simulink model "VCMGCM1962020b_v2"  (R2020b)
settings: Solver=FixedStepDiscrete  StartTime=0.0  StopTime=10.0  FixedStep=0.005  RelTol=1e-3  EnableMultiTasking=on
PreLoadFcn:
  | try, model_open; catch, disp('Error occurred while executing model pre-load callback: model_open.m'); disp('Please assure that the MATLAB working directory is set to the model directory before opening.'); end
InitFcn:
  | try, model_open; catch, end
undefined symbols (not defined in the file): Bridge, GCM, H, raptor_get_param_eval, raptor_get_safe_string, raptor_xcp_function
libraries: Blocks_lib x1165, Raptor_lib x665, simulink x62, VCM_lib x5
(part 21 of 23)

== system VCMGCM1962020b_v2/Fgnd/Control/Drive Inverter/Motor Torque Request/Driver Torque Request/Cruise Control/Setpoint ==
  Data : Inport
  Bus Creator : BusCreator  Inputs=3
  Bus Selector5 : BusSelector  OutputSignals=VirtualSensors.Spd.VehSpd [kph],VirtualSensors.Driver.CCOn [Bool],VirtualSensors.Driver.CCSetCst [Bool],VirtualSensors.Driver.CCRsmAcc [Bool]
  Enable : Subsystem
  Header : Blocks_lib/Header  width=Portrait  addtext=''
  Meas&Ovrd : Blocks_lib/Meas&Ovrd  nam='CCActv'  name_source=Parameter  view_as=Number  enum_struct={}  gain=1  min=-inf  max=inf  precision=''  units='Bool'  help='Cruise control active'  group=group
  Meas&Ovrd1 : Blocks_lib/Meas&Ovrd  nam='CCSetpt'  name_source=Parameter  view_as=Number  enum_struct={}  gain=1  min=-inf  max=inf  precision=''  units='kph'  help='Cruise control setpoint'  group=group
  Setpoint : Stateflow chart  TreatAsAtomicUnit=on
  SetptMnMx : Subsystem
  Standby : Subsystem
  raptor_adjustment : Raptor_lib/Data Storage/raptor_adjustment  paramName='CCTapTimeThr'  nameSource=Parameter  initValue=0 / samptime  dataType=uint16  storage=Calibration  calDispType=Number  calEnum={'Disabled', 'Enabled'}  calGain=samptime  calOffset=0  calMax=inf  calMin=-inf  calFormat=''  calUnit='sec'  calHelp='Cruise control tap time threshold'  calAccess=1  calFunction=group  calDispHeaders=off  calColHeaders={'Col1' 'Col2' 'Col3'}  calRowHeaders={'Row1' 'Row2' 'Row3'}
      settings: SourceProductName=Raptor
  raptor_adjustment1 : Raptor_lib/Data Storage/raptor_adjustment  paramName='CCDecDeltaMx'  nameSource=Parameter  initValue=0  dataType=double  storage=Calibration  calDispType=Number  calEnum={'Disabled', 'Enabled'}  calGain=1  calOffset=0  calMax=inf  calMin=-inf  calFormat=''  calUnit='kph'  calHelp='Cruise control decrement delta (between vehicle speed and setpoint) maximum'  calAccess=1  calFunction=group  calDispHeaders=off  calColHeaders={'Col1' 'Col2' 'Col3'}  calRowHeaders={'Row1' 'Row2' 'Row3'}
      settings: SourceProductName=Raptor
  raptor_adjustment2 : Raptor_lib/Data Storage/raptor_adjustment  paramName='CCTapInc'  nameSource=Parameter  initValue=0  dataType=double  storage=Calibration  calDispType=Number  calEnum={'Disabled', 'Enabled'}  calGain=1  calOffset=0  calMax=inf  calMin=-inf  calFormat=''  calUnit='kph'  calHelp='Cruise control tap increment'  calAccess=1  calFunction=group  calDispHeaders=off  calColHeaders={'Col1' 'Col2' 'Col3'}  calRowHeaders={'Row1' 'Row2' 'Row3'}
      settings: SourceProductName=Raptor
  raptor_adjustment3 : Raptor_lib/Data Storage/raptor_adjustment  paramName='CCAccRate'  nameSource=Parameter  initValue=0 * samptime  dataType=double  storage=Calibration  calDispType=Number  calEnum={'Disabled', 'Enabled'}  calGain=1/samptime  calOffset=0  calMax=inf  calMin=-inf  calFormat=''  calUnit='kph/s'  calHelp='Cruise control accelerate rate'  calAccess=1  calFunction=group  calDispHeaders=off  calColHeaders={'Col1' 'Col2' 'Col3'}  calRowHeaders={'Row1' 'Row2' 'Row3'}
      settings: SourceProductName=Raptor
  raptor_measurement : Raptor_lib/Data Storage/raptor_measurement  paramName='CCState'  nameSource=Parameter  calDispType=Number  calEnum={}  calGain=1  calOffset=0  calMax=inf  calMin=-inf  calFormat=''  calUnit='enum'  calHelp='Cruise control state'  calAccess=1  calFunction=group  calVisible=on
      settings: SourceProductName=Raptor
  Setpt : Outport  VectorParamsAs1DForOutWhenUnconnected=off
  wires:
  SetptMnMx/2(Mn) -> Setpoint/12(SetptMn)
  SetptMnMx/1(Mx) -> Setpoint/11(SetptMx)
  Setpoint/1(State) -> Bus Creator/1, raptor_measurement/1  "CCState [enum]"
  Meas&Ovrd1/1 -> Bus Creator/3
  Meas&Ovrd/1 -> Bus Creator/2
  raptor_adjustment1/1 -> Setpoint/8(DecDeltaMx)
  raptor_adjustment2/1 -> Setpoint/9(TapInc)
  Bus Creator/1 -> Setpt/1  "CCSetpt"
  Setpoint/2(Actv) -> Meas&Ovrd/1
  Setpoint/3(Setpt) -> Meas&Ovrd1/1
  raptor_adjustment/1 -> Setpoint/7(TapThr)
  Enable/1(Enbl) -> Setpoint/1(Enbl)
  raptor_adjustment3/1 -> Setpoint/10(AccInc)
  Standby/1(Stndby) -> Setpoint/2(Standby)
  Bus Selector5/2 -> Setpoint/4(On)  "<CCOn [Bool]>"
  Bus Selector5/3 -> Setpoint/5(SetCst)  "<CCSetCst [Bool]>"
  Bus Selector5/4 -> Setpoint/6(RsmAcc)  "<CCRsmAcc [Bool]>"
  Data/1 -> Enable/1(Data), Standby/1(Data), Bus Selector5/1, SetptMnMx/1(Data)
  Bus Selector5/1 -> Setpoint/3(Spd)  "<VehSpd [kph]>"

== system VCMGCM1962020b_v2/Fgnd/Control/Drive Inverter/Motor Torque Request/Driver Torque Request/Driveability/Rate Limit ==
  Data : Inport
  TrqReq : Inport  Port=2
  Bus Selector : BusSelector  OutputSignals=VirtualSensors.Spd.VehSpd [kph]
  Compare To Zero : simulink/Logic and Bit Operations/Compare To Zero  relop=<  OutDataTypeStr=boolean
  Gain : Gain  Gain=-1
  Header : Blocks_lib/Header  width=Portrait  addtext=''
  Multiport Switch : MultiPortSwitch  DataPortOrder=Zero-based contiguous  Inputs=2  zeroidx=on  InputSameDT=on
  Mux : Mux  Inputs=2
  Selector : Selector  InputPortWidth=2  IndexOptions=Index vector (dialog)  Indices=[2 1]  OutputSizes=1
  raptor_table_axis : Raptor_lib/Table Lookup/raptor_table_axis  dataName='VehSpd05IdxArr'  initValue=[1:05]  dataType=double  storage=Calibration  calVisible=on  calGain=1.0  calOffset=0  calMax=Inf  calMin=-Inf  calFormat='-1'  calUnit='kph'  calHelp='Index array'  calAccess=1  calFunction=group
      settings: SourceProductName=Raptor
  raptor_table_interpolate_1d : Raptor_lib/Table Lookup/raptor_table_interpolate_1d  dataName='DrvTrqReqRateLimIncTbl'  initValue=zeros(1,5)  dataType=double  storage=Calibration  adapt=off  adaptMode=Adapt between points  adaptOut=off  calVisible=on  calGain=1.0  calOffset=0.0  calMax=Inf  calMin=-Inf  calFormat='-1'  calUnit='Nm/s'  calHelp='Driver torque request rate limit (in increasing direction away from zero)'  calAccess=1  calFunction=group  measureEnable=on  mName='DrvTrqReqRateLimInc'
      settings: SourceProductName=Raptor
  raptor_table_interpolate_1d1 : Raptor_lib/Table Lookup/raptor_table_interpolate_1d  dataName='DrvTrqReqRateLimDecTbl'  initValue=zeros(1,5)  dataType=double  storage=Calibration  adapt=off  adaptMode=Adapt between points  adaptOut=off  calVisible=on  calGain=1.0  calOffset=0.0  calMax=Inf  calMin=-Inf  calFormat='-1'  calUnit='Nm/s'  calHelp='Driver torque request rate limit (in decreasing direction towards zero)'  calAccess=1  calFunction=group  measureEnable=on  mName='DrvTrqReqRateLimDec'
      settings: SourceProductName=Raptor
  Nm/s : Outport  VectorParamsAs1DForOutWhenUnconnected=off
  wires:
  Multiport Switch/1 -> Nm/s/1
  raptor_table_interpolate_1d1/1 -> Mux/2
  raptor_table_interpolate_1d/1 -> Mux/1
  Gain/1 -> Multiport Switch/3
  Selector/1 -> Gain/1
  Compare To Zero/1 -> Multiport Switch/1
  Data/1 -> Bus Selector/1
  Bus Selector/1 -> raptor_table_axis/1  "<VehSpd [kph]>"
  TrqReq/1 -> Compare To Zero/1
  raptor_table_axis/1 -> raptor_table_interpolate_1d/1, raptor_table_interpolate_1d1/1
  Mux/1 -> Selector/1, Multiport Switch/2

== system VCMGCM1962020b_v2/Fgnd/Control/Drive Inverter/Motor Torque Request/Driver Torque Request/Pedal Torque Request/APP When Two Pedal Driving ==
  Data : Inport
  Bus Selector : BusSelector  OutputSignals=VirtualSensors.Driver.BrkSw [Bool],VirtualSensors.Driver.APP [%]
  Header : Blocks_lib/Header  width=Portrait  addtext=''
  MinMax : MinMax  Inputs=2
  Multiport Switch : MultiPortSwitch  DataPortOrder=Zero-based contiguous  Inputs=2  zeroidx=on
  raptor_adjustment : Raptor_lib/Data Storage/raptor_adjustment  paramName='APPMxTwoPedalDrv'  nameSource=Parameter  initValue=0  dataType=double  storage=Calibration  calDispType=Number  calEnum={'False', 'True'}  calGain=1.0  calOffset=0.0  calMax=inf  calMin=-inf  calFormat='-1'  calUnit='%'  calHelp='APP maximum (when two pedal driving)'  calAccess=1  calFunction=group  calDispHeaders=off  calColHeaders={'Col1' 'Col2' 'Col3'}  calRowHeaders={'Row1' 'Row2' 'Row3'}
      settings: SourceProductName=Raptor
  % : Outport  VectorParamsAs1DForOutWhenUnconnected=off
  wires:
  Data/1 -> Bus Selector/1
  Multiport Switch/1 -> %/1
  Bus Selector/1 -> Multiport Switch/1  "<BrkSw [Bool]>"
  MinMax/1 -> Multiport Switch/3
  raptor_adjustment/1 -> MinMax/2
  Bus Selector/2 -> Multiport Switch/2, MinMax/1  "<APP [%]>"

== system VCMGCM1962020b_v2/Fgnd/Control/Drive Inverter/Motor Torque Request/Driver Torque Request/Pedal Torque Request/Apply Sign to Vehicle Speed ==
  Data : Inport
  Bus Selector : BusSelector  OutputSignals=VirtualSensors.Spd.VehDir [enum],Control.Mode.PRNDMode [enum],VirtualSensors.Spd.VehSpd [kph]
  CmprTo : Blocks_lib/CmprTo  op===  val='Rev'  enum=EnumLst.VehDir
  CmprTo1 : Blocks_lib/CmprTo  op===  val='Rev'  enum=EnumLst.PRNDMode
  Filt : Blocks_lib/Filt  nam='APPTrqReqMapVehSpdFiltTC'  group=group  samptime=samptime
  Gain : Gain  Gain=-1
  Header : Blocks_lib/Header  width=Portrait  addtext=''
  Logical Operator : Logic  Operator=XOR  AllPortsSameDT=off  OutDataTypeStr=boolean
  Multiport Switch : MultiPortSwitch  DataPortOrder=Zero-based contiguous  Inputs=2  zeroidx=on
  kph : Outport  VectorParamsAs1DForOutWhenUnconnected=off
  wires:
  CmprTo1/1 -> Logical Operator/2
  Logical Operator/1 -> Multiport Switch/1
  Bus Selector/2 -> CmprTo1/1  "<PRNDMode [enum]>"
  Bus Selector/3 -> Gain/1, Multiport Switch/2  "<VehSpd [kph]>"
  Gain/1 -> Multiport Switch/3
  Bus Selector/1 -> CmprTo/1  "<VehDir [enum]>"
  Multiport Switch/1 -> Filt/1
  Data/1 -> Bus Selector/1
  CmprTo/1 -> Logical Operator/1
  Filt/1 -> kph/1

== system VCMGCM1962020b_v2/Fgnd/Control/Drive Inverter/Motor Torque Request/Driver Torque Request/Pedal Torque Request/Creep Torque ==
  Data : Inport
  Bus Selector : BusSelector  OutputSignals=VirtualSensors.Driver.BrkSw [Bool],VirtualSensors.Spd.VehSpd [kph]
  Constant : Constant  Value=double(0)
  Header : Blocks_lib/Header  width=Portrait  addtext=''
  Multiport Switch : MultiPortSwitch  DataPortOrder=Zero-based contiguous  Inputs=2  zeroidx=on
  raptor_table_1d : Raptor_lib/Table Lookup/raptor_table_1d  dataName='CreepTrqReqTbl'  initValue=zeros(1,5)  dataType=double  storage=Calibration  initValueX=[1:5]  dataTypeXY=double  storageXY=Calibration  calVisible=on  showTable=on  calGain=1.0  calOffset=0.0  calMax=Inf  calMin=-Inf  calFormat='-1'  calUnit='Nm'  calHelp='Creep torque request'  showBreakpoint=on  dataNameX='VehSpdLo05IdxArr'  calGainX=1.0  calOffsetX=0.0  calMaxX=Inf  calMinX=-Inf  calFormatX='-1'  calUnitX='kph'  calHelpX='Index array'  calAccess=1  calFunction=group  measureEnable=on  mName='CreepTrqReq'
      settings: SourceProductName=Raptor
  Nm : Outport  VectorParamsAs1DForOutWhenUnconnected=off
  wires:
  Bus Selector/2 -> raptor_table_1d/1  "<VehSpd [kph]>"
  Constant/1 -> Multiport Switch/3
  Multiport Switch/1 -> Nm/1
  raptor_table_1d/1 -> Multiport Switch/2
  Data/1 -> Bus Selector/1
  Bus Selector/1 -> Multiport Switch/1  "<BrkSw [Bool]>"

== system VCMGCM1962020b_v2/Fgnd/Control/Drive Inverter/Motor Torque Request/Driver Torque Request/Vehicle Speed Limiter/Vehicle Speed Limit ==
  Header : Blocks_lib/Header  width=Portrait  addtext=''
  MinMax : MinMax  Inputs=2
  Multiport Switch : MultiPortSwitch  DataPortOrder=Zero-based contiguous  Inputs=2  zeroidx=on  InputSameDT=on
  raptor_adjustment : Raptor_lib/Data Storage/raptor_adjustment  paramName='VehSpdLim_cal'  nameSource=Parameter  initValue=0.00  dataType=double  storage=Calibration  calDispType=Number  calEnum={'False', 'True'}  calGain=1.0  calOffset=0.0  calMax=inf  calMin=-inf  calFormat='-1'  calUnit='kph'  calHelp='Vehicle speed limit'  calAccess=1  calFunction=group  calDispHeaders=off  calColHeaders={'Col1' 'Col2' 'Col3'}  calRowHeaders={'Row1' 'Row2' 'Row3'}
      settings: SourceProductName=Raptor
  raptor_adjustment1 : Raptor_lib/Data Storage/raptor_adjustment  paramName='VehSpdLimFault'  nameSource=Parameter  initValue=0.00  dataType=double  storage=Calibration  calDispType=Number  calEnum={'False', 'True'}  calGain=1.0  calOffset=0.0  calMax=inf  calMin=-inf  calFormat='-1'  calUnit='kph'  calHelp='Vehicle speed limit (if VehSpdLim fault action active)'  calAccess=1  calFunction=group  calDispHeaders=off  calColHeaders={'Col1' 'Col2' 'Col3'}  calRowHeaders={'Row1' 'Row2' 'Row3'}
      settings: SourceProductName=Raptor
  raptor_fault_action : Raptor_lib/Faults/raptor_fault_action  actionName='VehSpdLim'  calVisible=off  calAccess=1  calFunction='System | FaultManager | FaultAction'
      settings: SourceProductName=Raptor
  raptor_measurement : Raptor_lib/Data Storage/raptor_measurement  paramName='VehSpdLim'  nameSource=Parameter  calDispType=Number  calEnum={'Disabled', 'Enabled'}  calGain=1  calOffset=0  calMax=inf  calMin=-inf  calFormat=''  calUnit='kph'  calHelp='Vehicle speed limit'  calAccess=1  calFunction=group  calVisible=on
      settings: SourceProductName=Raptor
  kph : Outport  VectorParamsAs1DForOutWhenUnconnected=off
  wires:
  raptor_adjustment/1 -> MinMax/1, Multiport Switch/2
  MinMax/1 -> Multiport Switch/3
  Multiport Switch/1 -> kph/1, raptor_measurement/1
  raptor_adjustment1/1 -> MinMax/2
  raptor_fault_action/1 -> Multiport Switch/1

== system VCMGCM1962020b_v2/Fgnd/Control/Drive Inverter/Motor Torque Request/Inverter//Motor Limit & Request/Motor Torque Limit/CAN ==
  Data : Inport
  Bus Selector : BusSelector  OutputSignals=VirtualSensors.DrvInvtr.DrvMtrTrqLimMx [Nm],VirtualSensors.DrvInvtr.DrvMtrTrqLimMn [Nm]
  Header : Blocks_lib/Header  width=Portrait  addtext=''
  Mux : Mux  Inputs=2
  raptor_measurement : Raptor_lib/Data Storage/raptor_measurement  paramName=[mtrnam 'TrqLimCAN']  nameSource=Parameter  calDispType=Number  calEnum={'Disabled', 'Enabled'}  calGain=1  calOffset=0  calMax=inf  calMin=-inf  calFormat=''  calUnit='Nm'  calHelp='Motor torque limit (based on limits over CAN)'  calAccess=1  calFunction=group  calVisible=on
      settings: SourceProductName=Raptor
  Nm : Outport  VectorParamsAs1DForOutWhenUnconnected=off
  wires:
  Data/1 -> Bus Selector/1
  Bus Selector/2 -> Mux/2  "<DrvMtrTrqLimMn [Nm]>"
  Bus Selector/1 -> Mux/1  "<DrvMtrTrqLimMx [Nm]>"
  Mux/1 -> Nm/1, raptor_measurement/1

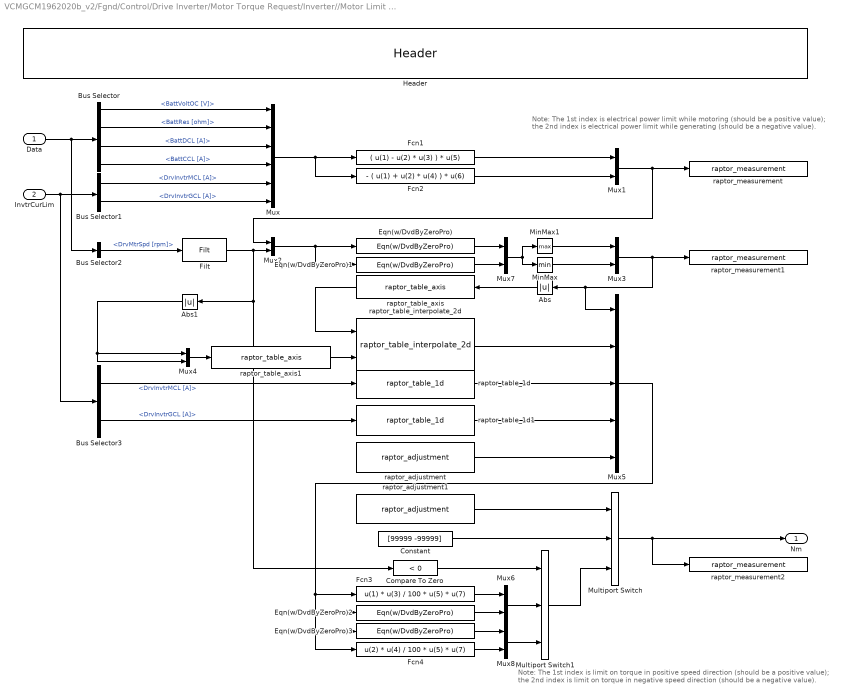
== system VCMGCM1962020b_v2/Fgnd/Control/Drive Inverter/Motor Torque Request/Inverter//Motor Limit & Request/Motor Torque Limit/Current Control ==
  note: Note:
      | The 1st index is electrical power limit while motoring (should be a positive value);
      | the 2nd index is electrical power limit while generating (should be a negative value).
  note: Note:
      | The 1st index is limit on torque in positive speed direction (should be a positive value);
      | the 2nd index is limit on torque in negative speed direction (should be a negative value).
  Data : Inport
  InvtrCurLim : Inport  Port=2
  Abs : Abs
  Abs1 : Abs
  Bus Selector : BusSelector  OutputSignals=VirtualSensors.Batt.BattVoltOC [V],VirtualSensors.Batt.BattRes [ohm],VirtualSensors.Batt.BattDCL [A],VirtualSensors.Batt.BattCCL [A]
  Bus Selector1 : BusSelector  OutputSignals=DrvInvtrMCL [A],DrvInvtrGCL [A]
  Bus Selector2 : BusSelector  OutputSignals=VirtualSensors.DrvInvtr.DrvMtrSpd [rpm]
  Bus Selector3 : BusSelector  OutputSignals=DrvInvtrMCL [A],DrvInvtrGCL [A]
  Compare To Zero : simulink/Logic and Bit Operations/Compare To Zero  relop=<  OutDataTypeStr=boolean
  Constant : Constant  Value=[99999 -99999]  OutDataTypeStr=double
  Eqn(w/DvdByZeroPro) : Blocks_lib/Eqn(w//DvdByZeroPro)  eqn='u(1) / (u(3) * 2 * pi / 60)'  dmn='(u(3) * 2 * pi / 60)'  dfltval=99999
  Eqn(w/DvdByZeroPro)1 : Blocks_lib/Eqn(w//DvdByZeroPro)  eqn='u(2) / (u(3) * 2 * pi / 60)'  dmn='(u(3) * 2 * pi / 60)'  dfltval=-99999
  Eqn(w/DvdByZeroPro)2 : Blocks_lib/Eqn(w//DvdByZeroPro)  eqn='u(2) / u(4) * 100 * u(6) * u(7)'  dmn='u(4)'  dfltval=0
  Eqn(w/DvdByZeroPro)3 : Blocks_lib/Eqn(w//DvdByZeroPro)  eqn='u(1) / u(3) * 100 * u(6) * u(7)'  dmn='u(3)'  dfltval=0
  Fcn1 : Fcn  Expr=( u(1) - u(2) * u(3) ) * u(5)
  Fcn2 : Fcn  Expr=- ( u(1) + u(2) * u(4) ) * u(6)
  Fcn3 : Fcn  Expr=u(1) * u(3) / 100 * u(5) * u(7)
  Fcn4 : Fcn  Expr=u(2) * u(4) / 100 * u(5) * u(7)
  Filt : Blocks_lib/Filt  nam=[invtrnam 'MtrEffMap' mtrnam 'SpdFiltTC']  group=group  samptime=samptime
  Header : Blocks_lib/Header  width=Portrait  addtext=''
  MinMax : MinMax
  MinMax1 : MinMax  Function=max
  Multiport Switch : MultiPortSwitch  DataPortOrder=Zero-based contiguous  Inputs=2  zeroidx=on  InputSameDT=on
  Multiport Switch1 : MultiPortSwitch  DataPortOrder=Zero-based contiguous  Inputs=2  zeroidx=on  InputSameDT=on
  Mux : Mux  Inputs=6
  Mux{1..4,6..8} (7 alike) : Mux  Inputs=2
  Mux5 : Mux  Inputs=5
  raptor_adjustment : Raptor_lib/Data Storage/raptor_adjustment  paramName=[mtrnam 'TrqLimCurMultp']  nameSource=Parameter  initValue=0  dataType=double  storage=Calibration  calDispType=Number  calEnum={}  calGain=1  calOffset=0  calMax=inf  calMin=-inf  calFormat=''  calUnit='multp'  calHelp='Motor torque limit (based on current limits) multiplier (to reduce or add factor of safety)'  calAccess=1  calFunction=group  calDispHeaders=off  calColHeaders={'Col1' 'Col2' 'Col3'}  calRowHeaders={'Row1' 'Row2' 'Row3'}
      settings: SourceProductName=Raptor
  raptor_adjustment1 : Raptor_lib/Data Storage/raptor_adjustment  paramName=[mtrnam 'TrqLimCurEnbl']  nameSource=Parameter  initValue=0  dataType=boolean  storage=Calibration  calDispType=Number  calEnum={'False', 'True'}  calGain=1  calOffset=0  calMax=inf  calMin=-inf  calFormat=''  calUnit='Bool'  calHelp='Motor torque limit (based on current limits) enable'  calAccess=1  calFunction=group  calDispHeaders=off  calColHeaders={'Col1' 'Col2' 'Col3'}  calRowHeaders={'Row1' 'Row2' 'Row3'}
      settings: SourceProductName=Raptor
  raptor_measurement : Raptor_lib/Data Storage/raptor_measurement  paramName=[invtrnam 'ElecPwrLim']  nameSource=Parameter  calDispType=Number  calEnum={'Disabled', 'Enabled'}  calGain=1/1000  calOffset=0  calMax=inf  calMin=-inf  calFormat=''  calUnit='kW'  calHelp='Inverter electrical power limit'  calAccess=1  calFunction=group  calVisible=on
      settings: SourceProductName=Raptor
  raptor_measurement1 : Raptor_lib/Data Storage/raptor_measurement  paramName=[invtrnam 'ElecTrqLim']  nameSource=Parameter  calDispType=Number  calEnum={'Disabled', 'Enabled'}  calGain=1  calOffset=0  calMax=inf  calMin=-inf  calFormat=''  calUnit='Nm'  calHelp='Inverter electrical torque limit (with 100% inverter/motor efficiency)'  calAccess=1  calFunction=group  calVisible=on
      settings: SourceProductName=Raptor
  raptor_measurement2 : Raptor_lib/Data Storage/raptor_measurement  paramName=[mtrnam 'TrqLimCur']  nameSource=Parameter  calDispType=Number  calEnum={'Disabled', 'Enabled'}  calGain=1  calOffset=0  calMax=inf  calMin=-inf  calFormat=''  calUnit='Nm'  calHelp='Motor torque limit (based on current limits)'  calAccess=1  calFunction=group  calVisible=on
      settings: SourceProductName=Raptor
  raptor_table_1d : Raptor_lib/Table Lookup/raptor_table_1d  dataName=[mtrnam 'TrqLimCurMultpInvtrMCLTbl']  initValue=zeros(1,7)  dataType=double  storage=Calibration  initValueX=[1:7]  dataTypeXY=double  storageXY=Calibration  calVisible=on  showTable=on  calGain=1.0  calOffset=0.0  calMax=Inf  calMin=-Inf  calFormat='-1'  calUnit='multp'  calHelp='Drive motor torque limit (based on current limits) multiplier (at low inverter MCL) (on positive torque only)'  showBreakpoint=on  dataNameX=[invtrnam 'MCLLo07IdxArr']  calGainX=1.0  calOffsetX=0.0  calMaxX=Inf  calMinX=-Inf  calFormatX='-1'  calUnitX='A'  calHelpX='Index array'  calAccess=1  calFunction=group  measureEnable=on  mName=[mtrnam 'TrqLimCurMultpInvtrMCL']
      settings: SourceProductName=Raptor
  raptor_table_1d1 : Raptor_lib/Table Lookup/raptor_table_1d  dataName=[mtrnam 'TrqLimCurMultpInvtrGCLTbl']  initValue=zeros(1,7)  dataType=double  storage=Calibration  initValueX=[1:7]  dataTypeXY=double  storageXY=Calibration  calVisible=on  showTable=on  calGain=1.0  calOffset=0.0  calMax=Inf  calMin=-Inf  calFormat='-1'  calUnit='multp'  calHelp='Drive motor torque limit (based on current limits) multiplier (at low inverter GCL) (on negative torque only)'  showBreakpoint=on  dataNameX=[invtrnam 'GCLLo07IdxArr']  calGainX=1.0  calOffsetX=0.0  calMaxX=Inf  calMinX=-Inf  calFormatX='-1'  calUnitX='A'  calHelpX='Index array'  calAccess=1  calFunction=group  measureEnable=on  mName=[mtrnam 'TrqLimCurMultpInvtrGCL']
      settings: SourceProductName=Raptor
  raptor_table_axis : Raptor_lib/Table Lookup/raptor_table_axis  dataName=[invtrnam 'ElecTrq11IdxArr']  initValue=[1:11]  dataType=double  storage=Calibration  calVisible=on  calGain=1  calOffset=0  calMax=inf  calMin=-inf  calFormat=''  calUnit='Nm'  calHelp='Index array'  calAccess=1  calFunction=group
      settings: SourceProductName=Raptor
  raptor_table_axis1 : Raptor_lib/Table Lookup/raptor_table_axis  dataName=[mtrnam 'Spd11IdxArr']  initValue=[1:11]  dataType=double  storage=Calibration  calVisible=on  calGain=1  calOffset=0  calMax=inf  calMin=-inf  calFormat=''  calUnit='rpm'  calHelp='Index array'  calAccess=1  calFunction=group
      settings: SourceProductName=Raptor
  raptor_table_interpolate_2d : Raptor_lib/Table Lookup/raptor_table_interpolate_2d  dataName=[invtrnam 'MtrEffMap']  initValue=zeros(11)  dataType=double  storage=Calibration  adapt=off  adaptMode=Adapt between points  adaptOut=off  calVisible=on  calGain=1  calOffset=0  calMax=inf  calMin=-inf  calFormat=''  calUnit='%'  calHelp='Inverter/motor efficiency'  calAccess=1  calFunction=group  measureEnable=off  mName=''
      settings: SourceProductName=Raptor
  Nm : Outport  VectorParamsAs1DForOutWhenUnconnected=off
  wires:
  Multiport Switch/1 -> raptor_measurement2/1, Nm/1
  Mux2/1 -> Eqn(w/DvdByZeroPro)1/1, Eqn(w/DvdByZeroPro)/1
  Mux3/1 -> raptor_measurement1/1, Mux5/1, Abs/1
  Mux/1 -> Fcn2/1, Fcn1/1
  Mux1/1 -> raptor_measurement/1, Mux2/1
  Bus Selector3/2 -> raptor_table_1d1/1  "<DrvInvtrGCL [A]>"
  Bus Selector3/1 -> raptor_table_1d/1  "<DrvInvtrMCL [A]>"
  Mux4/1 -> raptor_table_axis1/1
  Bus Selector/4 -> Mux/4  "<BattCCL [A]>"
  Bus Selector/3 -> Mux/3  "<BattDCL [A]>"
  Bus Selector1/1 -> Mux/5  "<DrvInvtrMCL [A]>"
  Bus Selector/2 -> Mux/2  "<BattRes [ohm]>"
  Bus Selector1/2 -> Mux/6  "<DrvInvtrGCL [A]>"
  Bus Selector/1 -> Mux/1  "<BattVoltOC [V]>"
  InvtrCurLim/1 -> Bus Selector1/1, Bus Selector3/1
  Data/1 -> Bus Selector2/1, Bus Selector/1
  raptor_table_axis1/1 -> raptor_table_interpolate_2d/2
  Abs/1 -> raptor_table_axis/1
  Eqn(w/DvdByZeroPro)2/1 -> Mux6/2
  Fcn3/1 -> Mux6/1
  MinMax/1 -> Mux3/2
  MinMax1/1 -> Mux3/1
  Mux5/1 -> Fcn4/1, Eqn(w/DvdByZeroPro)3/1, Eqn(w/DvdByZeroPro)2/1, Fcn3/1
  raptor_table_axis/1 -> raptor_table_interpolate_2d/1
  raptor_adjustment/1 -> Mux5/5
  raptor_table_interpolate_2d/1 -> Mux5/2
  Eqn(w/DvdByZeroPro)1/1 -> Mux7/2
  Eqn(w/DvdByZeroPro)/1 -> Mux7/1
  Bus Selector2/1 -> Filt/1  "<DrvMtrSpd [rpm]>"
  raptor_adjustment1/1 -> Multiport Switch/1
  Mux6/1 -> Multiport Switch1/2
  Constant/1 -> Multiport Switch/2
  Fcn1/1 -> Mux1/1
  Fcn2/1 -> Mux1/2
  Abs1/1 -> Mux4/2, Mux4/1
  Mux7/1 -> MinMax/1, MinMax1/1
  raptor_table_1d/1 -> Mux5/3
  raptor_table_1d1/1 -> Mux5/4
  Compare To Zero/1 -> Multiport Switch1/1
  Mux8/1 -> Multiport Switch1/3
  Eqn(w/DvdByZeroPro)3/1 -> Mux8/1
  Fcn4/1 -> Mux8/2
  Multiport Switch1/1 -> Multiport Switch/3
  Filt/1 -> Mux2/2, Compare To Zero/1, Abs1/1

== system VCMGCM1962020b_v2/Fgnd/Control/Drive Inverter/Motor Torque Request/Inverter//Motor Limit & Request/Motor Torque Limit/Derate Multiplier ==
  Data : Inport
  Bus Selector : BusSelector  OutputSignals=VirtualSensors.DrvInvtr.DrvInvtrTemp [degC],VirtualSensors.DrvInvtr.DrvMtrTemp [degC]
  Header : Blocks_lib/Header  width=Portrait  addtext=''
  Product : Product  InputSameDT=on  RndMeth=Zero  OutDataTypeStr=Inherit: Same as first input
  raptor_measurement : Raptor_lib/Data Storage/raptor_measurement  paramName=[mtrnam 'TrqLimMultp']  nameSource=Parameter  calDispType=Number  calEnum={'Disabled', 'Enabled'}  calGain=1  calOffset=0  calMax=inf  calMin=-inf  calFormat=''  calUnit='multp'  calHelp='Motor torque limit multiplier'  calAccess=1  calFunction=group  calVisible=on
      settings: SourceProductName=Raptor
  raptor_table_1d : Raptor_lib/Table Lookup/raptor_table_1d  dataName=[mtrnam 'TrqLimMultpInvtrTempTbl']  initValue=zeros(1,7)  dataType=double  storage=Calibration  initValueX=[1:7]  dataTypeXY=double  storageXY=Calibration  calVisible=on  showTable=on  calGain=1.0  calOffset=0.0  calMax=Inf  calMin=-Inf  calFormat='-1'  calUnit='multp'  calHelp='Motor torque limit multiplier (at high inverter temperature)'  showBreakpoint=on  dataNameX=[invtrnam 'TempHi07IdxArr']  calGainX=1.0  calOffsetX=0.0  calMaxX=Inf  calMinX=-Inf  calFormatX='-1'  calUnitX='degC'  calHelpX='Index array'  calAccess=1  calFunction=group  measureEnable=on  mName=[mtrnam 'TrqLimMultpInvtrTemp']
      settings: SourceProductName=Raptor
  raptor_table_1d1 : Raptor_lib/Table Lookup/raptor_table_1d  dataName=[mtrnam 'TrqLimMultpMtrTempTbl']  initValue=zeros(1,7)  dataType=double  storage=Calibration  initValueX=[1:7]  dataTypeXY=double  storageXY=Calibration  calVisible=on  showTable=on  calGain=1.0  calOffset=0.0  calMax=Inf  calMin=-Inf  calFormat='-1'  calUnit='multp'  calHelp='Motor torque limit multiplier (at high motor temperature)'  showBreakpoint=on  dataNameX=[mtrnam 'TempHi07IdxArr']  calGainX=1.0  calOffsetX=0.0  calMaxX=Inf  calMinX=-Inf  calFormatX='-1'  calUnitX='degC'  calHelpX='Index array'  calAccess=1  calFunction=group  measureEnable=on  mName=[mtrnam 'TrqLimMultpMtrTemp']
      settings: SourceProductName=Raptor
  multp : Outport  VectorParamsAs1DForOutWhenUnconnected=off
  wires:
  Data/1 -> Bus Selector/1
  Bus Selector/1 -> raptor_table_1d/1  "<DrvInvtrTemp [degC]>"
  raptor_table_1d/1 -> Product/1
  Bus Selector/2 -> raptor_table_1d1/1  "<DrvMtrTemp [degC]>"
  raptor_table_1d1/1 -> Product/2
  Product/1 -> multp/1, raptor_measurement/1

== system VCMGCM1962020b_v2/Fgnd/Control/Drive Inverter/Motor Torque Request/Inverter//Motor Limit & Request/Motor Torque Request/Gearbox Preload ==
  note: Note: The gearbox is preloaded in the correct direction upon entering Reverse or Drive or
      | when zero torque is crossed from the regen direction (eg, when coasting to a stop).
      | Then, the output torque request is no less than the preload torque until the
      | input torque request exceeds the preload torque in the opposite direction.
  Data : Inport
  TrqReq : Inport  Port=2
  Fcn : Fcn  Expr=u(1) - 0.001
  Fcn1 : Fcn  Expr=u(1) + 0.001
  Header : Blocks_lib/Header  width=Portrait  addtext=''
  MinMax : MinMax
  MinMax1 : MinMax  Function=max
  MinMax2 : MinMax  Function=max  Inputs=2
  MinMax3 : MinMax  Function=max
  MinMax4 : MinMax  Inputs=2
  MinMax5 : MinMax
  Multiport Switch : MultiPortSwitch  DataPortOrder=Zero-based contiguous  zeroidx=on
  Multiport Switch1 : MultiPortSwitch  DataPortOrder=Zero-based contiguous  Inputs=2  zeroidx=on
  Preload Initialize : Subsystem
  RelOp(w/Hyst) : Blocks_lib/RelOp(w//Hyst)  relop=<=
  raptor_adjustment : Raptor_lib/Data Storage/raptor_adjustment  paramName=[mtrnam 'GearPreloadTrq']  nameSource=Parameter  initValue=[0 0]  dataType=double  storage=Calibration  calDispType=Number  calEnum={'False', 'True'}  calGain=1.0  calOffset=0.0  calMax=inf  calMin=-inf  calFormat=''  calUnit='Nm'  calHelp='Motor gearbox preload torqe (to mitigate gearbox backlash)'  calAccess=1  calFunction=group  calDispHeaders=off  calColHeaders={'Col1' 'Col2' 'Col3'}  calRowHeaders={'Row1' 'Row2' 'Row3'}
      settings: SourceProductName=Raptor
  Nm : Outport  VectorParamsAs1DForOutWhenUnconnected=off
  wires:
  Data/1 -> Preload Initialize/1(Data)
  MinMax2/1 -> Multiport Switch1/2
  Multiport Switch/1 -> RelOp(w/Hyst)/1, MinMax2/1, MinMax4/1
  MinMax5/1 -> MinMax4/2
  MinMax3/1 -> MinMax2/2
  MinMax4/1 -> Multiport Switch1/3
  RelOp(w/Hyst)/1 -> Multiport Switch1/1
  Fcn1/1 -> Multiport Switch/4
  Fcn/1 -> Multiport Switch/3
  Preload Initialize/1(enum) -> Multiport Switch/1
  MinMax1/1 -> Fcn1/1
  TrqReq/1 -> Multiport Switch/2, Preload Initialize/2(TrqReq)
  MinMax/1 -> Fcn/1
  Multiport Switch1/1 -> Nm/1
  raptor_adjustment/1 -> MinMax/1, MinMax1/1, RelOp(w/Hyst)/2, MinMax3/1, MinMax5/1

== system VCMGCM1962020b_v2/Fgnd/Control/Drive Inverter/Motor Torque Request/Inverter//Motor Limit & Request/Motor Torque Request/Rate Limit ==
  EnblReq : Inport
  TrqReq1/z : Inport  Port=2
  TrqReq : Inport  Port=3
  Abs : Abs
  Compare To Zero : simulink/Logic and Bit Operations/Compare To Zero  relop=<  OutDataTypeStr=boolean
  Gain : Gain  Gain=-1
  Header : Blocks_lib/Header  width=Portrait  addtext=''
  Logical Operator : Logic  Operator=NOT  AllPortsSameDT=off  OutDataTypeStr=boolean
  Multiport Switch : MultiPortSwitch  DataPortOrder=Zero-based contiguous  Inputs=2  zeroidx=on  InputSameDT=on
  Mux : Mux  Inputs=2
  RateLim : Subsystem  mask(RateLim){samptime=samptime}
      mask prompts: samptime "Sample Time (sec)"
      mask Display:
      | plot([0.5 0.6], [0.1 0.9]);
      | plot([0.55 0.55], [0.1 0.9]);
      | plot([0.4 0.7], [0.5 0.5]);
  Selector : Selector  InputPortWidth=2  IndexOptions=Index vector (dialog)  Indices=[2 1]  OutputSizes=1
  raptor_table_axis : Raptor_lib/Table Lookup/raptor_table_axis  dataName=[mtrnam 'TrqReq05IdxArr']  initValue=[1:5]  dataType=double  storage=Calibration  calVisible=on  calGain=1.0  calOffset=0  calMax=Inf  calMin=-Inf  calFormat='-1'  calUnit='Nm'  calHelp='Index array'  calAccess=1  calFunction=group
      settings: SourceProductName=Raptor
  raptor_table_interpolate_1d : Raptor_lib/Table Lookup/raptor_table_interpolate_1d  dataName=[mtrnam 'TrqReqRateLimIncTbl']  initValue=zeros(1,5)  dataType=double  storage=Calibration  adapt=off  adaptMode=Adapt between points  adaptOut=off  calVisible=on  calGain=1.0  calOffset=0.0  calMax=Inf  calMin=-Inf  calFormat='-1'  calUnit='Nm/s'  calHelp='Motor torque request rate limit (in increasing direction away from zero)'  calAccess=1  calFunction=group  measureEnable=on  mName=[mtrnam 'TrqReqRateLimInc']
      settings: SourceProductName=Raptor
  raptor_table_interpolate_1d1 : Raptor_lib/Table Lookup/raptor_table_interpolate_1d  dataName=[mtrnam 'TrqReqRateLimDecTbl']  initValue=zeros(1,5)  dataType=double  storage=Calibration  adapt=off  adaptMode=Adapt between points  adaptOut=off  calVisible=on  calGain=1.0  calOffset=0.0  calMax=Inf  calMin=-Inf  calFormat='-1'  calUnit='Nm/s'  calHelp='Motor torque request rate limit (in decreasing direction towards zero)'  calAccess=1  calFunction=group  measureEnable=on  mName=[mtrnam 'TrqReqRateLimDec']
      settings: SourceProductName=Raptor
  Nm : Outport  VectorParamsAs1DForOutWhenUnconnected=off
  wires:
  Logical Operator/1 -> RateLim/2(Rst)
  Multiport Switch/1 -> RateLim/4("[+R -R]")
  TrqReq/1 -> RateLim/3(In)
  EnblReq/1 -> Logical Operator/1
  RateLim/1(Out) -> Nm/1
  raptor_table_axis/1 -> raptor_table_interpolate_1d/1, raptor_table_interpolate_1d1/1
  Abs/1 -> raptor_table_axis/1
  TrqReq1/z/1 -> Compare To Zero/1, RateLim/1(Prev), Abs/1
  Selector/1 -> Gain/1
  raptor_table_interpolate_1d/1 -> Mux/1
  Compare To Zero/1 -> Multiport Switch/1
  raptor_table_interpolate_1d1/1 -> Mux/2
  Gain/1 -> Multiport Switch/3
  Mux/1 -> Selector/1, Multiport Switch/2

== system VCMGCM1962020b_v2/Fgnd/Control/Modes/Startup & Shutdown/HV System Disable/Flash Started/UDS Msg Rxd ==
  f : TriggerPort  TriggerType=function-call  VariantControl=Variant  PortDimensions=1
  Constant : Constant  Value=boolean(1)
  Header : Blocks_lib/Header  width=Portrait  addtext=''
  raptor_data_def : Raptor_lib/Data Storage/raptor_data_def  dataName='VCMFlashStarted'  initValue=0  dataType=boolean  storage=Volatile (RAM)  calVisible=on  calType=Measurement  calDispType=Number  calEnum={'False', 'True'}  calGain=1.0  calOffset=0  calMin=-inf  calMax=inf  calFormat='-1'  calUnit='Bool'  calHelp='VCM flash started'  calAccess=1  calFunction=group  calDispHeaders=off  calColHeaders={'Col1' 'Col2' 'Col3'}  calRowHeaders={'Row1' 'Row2' 'Row3'}
      settings: SourceProductName=Raptor
  raptor_data_write : Raptor_lib/Data Storage/raptor_data_write  dataName='VCMFlashStarted'  dataShape=Scalar  idxSource=Input Port  idxRow=1  idxCol=1
      settings: SourceProductName=Raptor
  wires:
  Constant/1 -> raptor_data_write/1

== system VCMGCM1962020b_v2/Fgnd/Sensors/CAN/Inverter/EM2_InvTemp/EM2InvTemp/CANRxFieldSingleFloat ==
  note: Note:
      | The field is considered valid if its corresponding message is valid (ie, not timed out).
  In : Inport
  BusCreator : BusCreator  Inputs=2
  Header : Blocks_lib/Header  width=Portrait  addtext=''
  Meas&Ovrd : Blocks_lib/Meas&Ovrd  nam=[nam 'Vld']  name_source=Parameter  view_as=Number  enum_struct={}  gain=1  min=-inf  max=inf  precision=''  units='Bool'  help='CAN field valid (no message timeout)'  group='Diagnostics | Data Validity'
  Meas&Ovrd1 : Blocks_lib/Meas&Ovrd  nam=nam  name_source=Parameter  view_as=Number  enum_struct=enum  gain=1  min=-inf  max=inf  precision=''  units=units  help='CAN field rx'  group=['Sensors | CAN | ' msgnam]
  Multiport Switch : MultiPortSwitch  DataPortOrder=Zero-based contiguous  Inputs=2  zeroidx=on  InputSameDT=on
  Signal Specification : SignalSpecification  OutDataTypeStr=double
  raptor_adjustment : Raptor_lib/Data Storage/raptor_adjustment  paramName=[nam 'DfltVal']  nameSource=Parameter  initValue=0  dataType=Inherit via back propagation  storage=Calibration  calDispType=Number  calEnum=enum  calGain=1  calOffset=0  calMax=inf  calMin=-inf  calFormat=''  calUnit=units  calHelp='Default value when CAN field invalid'  calAccess=1  calFunction='Diagnostics | Default Values'  calDispHeaders=off  calColHeaders={'Col1' 'Col2' 'Col3'}  calRowHeaders={'Row1' 'Row2' 'Row3'}
      settings: SourceProductName=Raptor
  raptor_data_read : Raptor_lib/Data Storage/raptor_data_read  dataName=[msgnam 'MsgVld']  dataShape=Scalar  idxSource=Input  idxRow=1  idxCol=1
      settings: SourceProductName=Raptor
  Out : Outport  VectorParamsAs1DForOutWhenUnconnected=off
  wires:
  Meas&Ovrd1/1 -> BusCreator/2
  BusCreator/1 -> Out/1  "EM2_InverterBridgeMaxTemp"
  Meas&Ovrd/1 -> BusCreator/1
  raptor_data_read/1 -> Multiport Switch/1, Meas&Ovrd/1
  In/1 -> Signal Specification/1
  Signal Specification/1 -> Multiport Switch/3
  raptor_adjustment/1 -> Multiport Switch/2
  Multiport Switch/1 -> Meas&Ovrd1/1

== system VCMGCM1962020b_v2/Fgnd/Sensors/CAN/Inverter/EM2_InvTemp/EM2MtrTemp/CANRxFieldSingleFloat ==
  note: Note:
      | The field is considered valid if its corresponding message is valid (ie, not timed out).
  In : Inport
  BusCreator : BusCreator  Inputs=2
  Header : Blocks_lib/Header  width=Portrait  addtext=''
  Meas&Ovrd : Blocks_lib/Meas&Ovrd  nam=[nam 'Vld']  name_source=Parameter  view_as=Number  enum_struct={}  gain=1  min=-inf  max=inf  precision=''  units='Bool'  help='CAN field valid (no message timeout)'  group='Diagnostics | Data Validity'
  Meas&Ovrd1 : Blocks_lib/Meas&Ovrd  nam=nam  name_source=Parameter  view_as=Number  enum_struct=enum  gain=1  min=-inf  max=inf  precision=''  units=units  help='CAN field rx'  group=['Sensors | CAN | ' msgnam]
  Multiport Switch : MultiPortSwitch  DataPortOrder=Zero-based contiguous  Inputs=2  zeroidx=on  InputSameDT=on
  Signal Specification : SignalSpecification  OutDataTypeStr=double
  raptor_adjustment : Raptor_lib/Data Storage/raptor_adjustment  paramName=[nam 'DfltVal']  nameSource=Parameter  initValue=0  dataType=Inherit via back propagation  storage=Calibration  calDispType=Number  calEnum=enum  calGain=1  calOffset=0  calMax=inf  calMin=-inf  calFormat=''  calUnit=units  calHelp='Default value when CAN field invalid'  calAccess=1  calFunction='Diagnostics | Default Values'  calDispHeaders=off  calColHeaders={'Col1' 'Col2' 'Col3'}  calRowHeaders={'Row1' 'Row2' 'Row3'}
      settings: SourceProductName=Raptor
  raptor_data_read : Raptor_lib/Data Storage/raptor_data_read  dataName=[msgnam 'MsgVld']  dataShape=Scalar  idxSource=Input  idxRow=1  idxCol=1
      settings: SourceProductName=Raptor
  Out : Outport  VectorParamsAs1DForOutWhenUnconnected=off
  wires:
  Meas&Ovrd1/1 -> BusCreator/2
  BusCreator/1 -> Out/1  "EM2_MotorSensorTemp"
  Meas&Ovrd/1 -> BusCreator/1
  raptor_data_read/1 -> Multiport Switch/1, Meas&Ovrd/1
  In/1 -> Signal Specification/1
  Signal Specification/1 -> Multiport Switch/3
  raptor_adjustment/1 -> Multiport Switch/2
  Multiport Switch/1 -> Meas&Ovrd1/1

== system VCMGCM1962020b_v2/Fgnd/Sensors/CAN/Inverter/EM3_DCV/EM3DCv/CANRxFieldSingleFloat ==
  note: Note:
      | The field is considered valid if its corresponding message is valid (ie, not timed out).
  In : Inport
  BusCreator : BusCreator  Inputs=2
  Header : Blocks_lib/Header  width=Portrait  addtext=''
  Meas&Ovrd : Blocks_lib/Meas&Ovrd  nam=[nam 'Vld']  name_source=Parameter  view_as=Number  enum_struct={}  gain=1  min=-inf  max=inf  precision=''  units='Bool'  help='CAN field valid (no message timeout)'  group='Diagnostics | Data Validity'
  Meas&Ovrd1 : Blocks_lib/Meas&Ovrd  nam=nam  name_source=Parameter  view_as=Number  enum_struct=enum  gain=1  min=-inf  max=inf  precision=''  units=units  help='CAN field rx'  group=['Sensors | CAN | ' msgnam]
  Multiport Switch : MultiPortSwitch  DataPortOrder=Zero-based contiguous  Inputs=2  zeroidx=on  InputSameDT=on
  Signal Specification : SignalSpecification  OutDataTypeStr=double
  raptor_adjustment : Raptor_lib/Data Storage/raptor_adjustment  paramName=[nam 'DfltVal']  nameSource=Parameter  initValue=0  dataType=Inherit via back propagation  storage=Calibration  calDispType=Number  calEnum=enum  calGain=1  calOffset=0  calMax=inf  calMin=-inf  calFormat=''  calUnit=units  calHelp='Default value when CAN field invalid'  calAccess=1  calFunction='Diagnostics | Default Values'  calDispHeaders=off  calColHeaders={'Col1' 'Col2' 'Col3'}  calRowHeaders={'Row1' 'Row2' 'Row3'}
      settings: SourceProductName=Raptor
  raptor_data_read : Raptor_lib/Data Storage/raptor_data_read  dataName=[msgnam 'MsgVld']  dataShape=Scalar  idxSource=Input  idxRow=1  idxCol=1
      settings: SourceProductName=Raptor
  Out : Outport  VectorParamsAs1DForOutWhenUnconnected=off
  wires:
  Meas&Ovrd1/1 -> BusCreator/2
  BusCreator/1 -> Out/1  "EM3_InverterDcV"
  Meas&Ovrd/1 -> BusCreator/1
  raptor_data_read/1 -> Multiport Switch/1, Meas&Ovrd/1
  In/1 -> Signal Specification/1
  Signal Specification/1 -> Multiport Switch/3
  raptor_adjustment/1 -> Multiport Switch/2
  Multiport Switch/1 -> Meas&Ovrd1/1

== system VCMGCM1962020b_v2/Fgnd/Sensors/CAN/Inverter/EM3_DCV/EM3PhCur/CANRxFieldSingleFloat ==
  note: Note:
      | The field is considered valid if its corresponding message is valid (ie, not timed out).
  In : Inport
  BusCreator : BusCreator  Inputs=2
  Header : Blocks_lib/Header  width=Portrait  addtext=''
  Meas&Ovrd : Blocks_lib/Meas&Ovrd  nam=[nam 'Vld']  name_source=Parameter  view_as=Number  enum_struct={}  gain=1  min=-inf  max=inf  precision=''  units='Bool'  help='CAN field valid (no message timeout)'  group='Diagnostics | Data Validity'
  Meas&Ovrd1 : Blocks_lib/Meas&Ovrd  nam=nam  name_source=Parameter  view_as=Number  enum_struct=enum  gain=1  min=-inf  max=inf  precision=''  units=units  help='CAN field rx'  group=['Sensors | CAN | ' msgnam]
  Multiport Switch : MultiPortSwitch  DataPortOrder=Zero-based contiguous  Inputs=2  zeroidx=on  InputSameDT=on
  Signal Specification : SignalSpecification  OutDataTypeStr=double
  raptor_adjustment : Raptor_lib/Data Storage/raptor_adjustment  paramName=[nam 'DfltVal']  nameSource=Parameter  initValue=0  dataType=Inherit via back propagation  storage=Calibration  calDispType=Number  calEnum=enum  calGain=1  calOffset=0  calMax=inf  calMin=-inf  calFormat=''  calUnit=units  calHelp='Default value when CAN field invalid'  calAccess=1  calFunction='Diagnostics | Default Values'  calDispHeaders=off  calColHeaders={'Col1' 'Col2' 'Col3'}  calRowHeaders={'Row1' 'Row2' 'Row3'}
      settings: SourceProductName=Raptor
  raptor_data_read : Raptor_lib/Data Storage/raptor_data_read  dataName=[msgnam 'MsgVld']  dataShape=Scalar  idxSource=Input  idxRow=1  idxCol=1
      settings: SourceProductName=Raptor
  Out : Outport  VectorParamsAs1DForOutWhenUnconnected=off
  wires:
  Meas&Ovrd1/1 -> BusCreator/2
  BusCreator/1 -> Out/1  "EM3_PhaseAmpsRms"
  Meas&Ovrd/1 -> BusCreator/1
  raptor_data_read/1 -> Multiport Switch/1, Meas&Ovrd/1
  In/1 -> Signal Specification/1
  Signal Specification/1 -> Multiport Switch/3
  raptor_adjustment/1 -> Multiport Switch/2
  Multiport Switch/1 -> Meas&Ovrd1/1

== system VCMGCM1962020b_v2/Fgnd/Sensors/CAN/Inverter/EM4_Spd/EM4Spd/CANRxFieldSingleFloat ==
  note: Note:
      | The field is considered valid if its corresponding message is valid (ie, not timed out).
  In : Inport
  BusCreator : BusCreator  Inputs=2
  Header : Blocks_lib/Header  width=Portrait  addtext=''
  Meas&Ovrd : Blocks_lib/Meas&Ovrd  nam=[nam 'Vld']  name_source=Parameter  view_as=Number  enum_struct={}  gain=1  min=-inf  max=inf  precision=''  units='Bool'  help='CAN field valid (no message timeout)'  group='Diagnostics | Data Validity'
  Meas&Ovrd1 : Blocks_lib/Meas&Ovrd  nam=nam  name_source=Parameter  view_as=Number  enum_struct=enum  gain=1  min=-inf  max=inf  precision=''  units=units  help='CAN field rx'  group=['Sensors | CAN | ' msgnam]
  Multiport Switch : MultiPortSwitch  DataPortOrder=Zero-based contiguous  Inputs=2  zeroidx=on  InputSameDT=on
  Signal Specification : SignalSpecification  OutDataTypeStr=double
  raptor_adjustment : Raptor_lib/Data Storage/raptor_adjustment  paramName=[nam 'DfltVal']  nameSource=Parameter  initValue=0  dataType=Inherit via back propagation  storage=Calibration  calDispType=Number  calEnum=enum  calGain=1  calOffset=0  calMax=inf  calMin=-inf  calFormat=''  calUnit=units  calHelp='Default value when CAN field invalid'  calAccess=1  calFunction='Diagnostics | Default Values'  calDispHeaders=off  calColHeaders={'Col1' 'Col2' 'Col3'}  calRowHeaders={'Row1' 'Row2' 'Row3'}
      settings: SourceProductName=Raptor
  raptor_data_read : Raptor_lib/Data Storage/raptor_data_read  dataName=[msgnam 'MsgVld']  dataShape=Scalar  idxSource=Input  idxRow=1  idxCol=1
      settings: SourceProductName=Raptor
  Out : Outport  VectorParamsAs1DForOutWhenUnconnected=off
  wires:
  Meas&Ovrd1/1 -> BusCreator/2
  BusCreator/1 -> Out/1  "EM4_SpdAct"
  Meas&Ovrd/1 -> BusCreator/1
  raptor_data_read/1 -> Multiport Switch/1, Meas&Ovrd/1
  In/1 -> Signal Specification/1
  Signal Specification/1 -> Multiport Switch/3
  raptor_adjustment/1 -> Multiport Switch/2
  Multiport Switch/1 -> Meas&Ovrd1/1

== system VCMGCM1962020b_v2/Fgnd/Sensors/CAN/Inverter/EM4_Spd/EM4Torq/CANRxFieldSingleFloat ==
  note: Note:
      | The field is considered valid if its corresponding message is valid (ie, not timed out).
  In : Inport
  BusCreator : BusCreator  Inputs=2
  Header : Blocks_lib/Header  width=Portrait  addtext=''
  Meas&Ovrd : Blocks_lib/Meas&Ovrd  nam=[nam 'Vld']  name_source=Parameter  view_as=Number  enum_struct={}  gain=1  min=-inf  max=inf  precision=''  units='Bool'  help='CAN field valid (no message timeout)'  group='Diagnostics | Data Validity'
  Meas&Ovrd1 : Blocks_lib/Meas&Ovrd  nam=nam  name_source=Parameter  view_as=Number  enum_struct=enum  gain=1  min=-inf  max=inf  precision=''  units=units  help='CAN field rx'  group=['Sensors | CAN | ' msgnam]
  Multiport Switch : MultiPortSwitch  DataPortOrder=Zero-based contiguous  Inputs=2  zeroidx=on  InputSameDT=on
  Signal Specification : SignalSpecification  OutDataTypeStr=double
  raptor_adjustment : Raptor_lib/Data Storage/raptor_adjustment  paramName=[nam 'DfltVal']  nameSource=Parameter  initValue=0  dataType=Inherit via back propagation  storage=Calibration  calDispType=Number  calEnum=enum  calGain=1  calOffset=0  calMax=inf  calMin=-inf  calFormat=''  calUnit=units  calHelp='Default value when CAN field invalid'  calAccess=1  calFunction='Diagnostics | Default Values'  calDispHeaders=off  calColHeaders={'Col1' 'Col2' 'Col3'}  calRowHeaders={'Row1' 'Row2' 'Row3'}
      settings: SourceProductName=Raptor
  raptor_data_read : Raptor_lib/Data Storage/raptor_data_read  dataName=[msgnam 'MsgVld']  dataShape=Scalar  idxSource=Input  idxRow=1  idxCol=1
      settings: SourceProductName=Raptor
  Out : Outport  VectorParamsAs1DForOutWhenUnconnected=off
  wires:
  Meas&Ovrd1/1 -> BusCreator/2
  BusCreator/1 -> Out/1  "EM4_TorqAct"
  Meas&Ovrd/1 -> BusCreator/1
  raptor_data_read/1 -> Multiport Switch/1, Meas&Ovrd/1
  In/1 -> Signal Specification/1
  Signal Specification/1 -> Multiport Switch/3
  raptor_adjustment/1 -> Multiport Switch/2
  Multiport Switch/1 -> Meas&Ovrd1/1

== system VCMGCM1962020b_v2/Fgnd/Virtual Sensors/PDU/HVBusVolt/HV Bus Voltage/Diag/EvalDiag ==
  V : Inport
  Reset : EnablePort  StatesWhenEnabling=reset
  Abs : Abs
  Add1 : Sum  Inputs=+-
  FltRngTmr : Blocks_lib/FltRngTmr  nam=[nam 'XChk']  relop=>  threshnam=[nam 'XChkThr']  typ=double  units='V'  help='Cross-check fault threshold'  tmrth_nam=[nam 'XChkTimeThr']  tmrth_typ=uint16  tmrth_help='Cross-check fault time threshold'  samptime=samptime  group='Diagnostics | System'
  Header : Blocks_lib/Header  width=Portrait  addtext=''
  MinMax : MinMax  Function=max
  Mux : Mux  Inputs=2
  raptor_data_read1 : Raptor_lib/Data Storage/raptor_data_read  dataName=[nam 'Mx']  dataShape=Scalar  idxSource=Input  idxRow=1  idxCol=1
      settings: SourceProductName=Raptor
  raptor_data_read2 : Raptor_lib/Data Storage/raptor_data_read  dataName=[nam 'Mn']  dataShape=Scalar  idxSource=Input  idxRow=1  idxCol=1
      settings: SourceProductName=Raptor
  wires:
  V/1 -> Add1/1
  raptor_data_read1/1 -> Mux/1
  Add1/1 -> Abs/1
  Abs/1 -> MinMax/1
  raptor_data_read2/1 -> Mux/2
  Mux/1 -> Add1/2
  MinMax/1 -> FltRngTmr/1

== system VCMGCM1962020b_v2/Fgnd/Virtual Sensors/PDU/HVBusVolt/HV Bus Voltage/Sum, Max, Min/Data Vectors ==
  note: Note: HV bus voltage readings available from:
      | - Drive inverter
      | -DCDC
      | - Charger
  Data : Inport
  AND : Logic  AllPortsSameDT=off  OutDataTypeStr=boolean
  AND1 : Logic  AllPortsSameDT=off  OutDataTypeStr=boolean
  Bus Selector : BusSelector  OutputSignals=VirtualSensors.DrvInvtr.DrvInvtrVolt [V],VirtualSensors.DCDC.DCDCInptVolt [V],VirtualSensors.Chgr.OnBoard.OnBoardChgrDCVolt [V]
  Bus Selector1 : BusSelector  OutputSignals=VirtualSensors.DrvInvtr.DrvInvtrVoltVld [Bool],Sensors.CAN.DCDC.DCDCConverterInputOutput.DCDCInputVoltage.DCDCInputVoltageVld [Bool],Sensors.Sensors.Other.DCDCCntrClosed.DCDCCntrClosed [Bool],Sensors.CAN.OnBoardChgr.ChgrCCSA.ChgrChrgr_Out_volt.ChgrChrgr_Out_voltVld [Bool],Sensors.Sensors.Other.ChrgrCntrClosed.ChrgrCntrClosed [Bool]
  Header : Blocks_lib/Header  width=Portrait  addtext=''
  Mux : Mux  Inputs=3
  Mux1 : Mux  Inputs=3
  V : Outport  VectorParamsAs1DForOutWhenUnconnected=off
  Vld : Outport  Port=2  VectorParamsAs1DForOutWhenUnconnected=off
  wires:
  Mux1/1 -> Vld/1
  Mux/1 -> V/1
  Bus Selector/2 -> Mux/2  "<DCDCInptVolt [V]>"
  Bus Selector/3 -> Mux/3  "<OnBoardChgrDCVolt [V]>"
  Data/1 -> Bus Selector1/1, Bus Selector/1
  Bus Selector/1 -> Mux/1  "<DrvInvtrVolt [V]>"
  Bus Selector1/1 -> Mux1/1  "<DrvInvtrVoltVld [Bool]>"
  AND1/1 -> Mux1/3
  AND/1 -> Mux1/2
  Bus Selector1/2 -> AND/1  "<DCDCInputVoltageVld [Bool]>"
  Bus Selector1/3 -> AND/2  "<DCDCCntrClosed [Bool]>"
  Bus Selector1/4 -> AND1/1  "<ChgrChrgr_Out_voltVld [Bool]>"
  Bus Selector1/5 -> AND1/2  "<ChrgrCntrClosed [Bool]>"

== system VCMGCM1962020b_v2/Fgnd/Virtual Sensors/PDU/HVBusVolt/HV Bus Voltage/Sum, Max, Min/Loop ==
  V : Inport
  Vld : Inport  Port=2
  N : Inport  Port=3
  Data Valid : Subsystem
  For Iterator : ForIterator  IterationSource=external  IterationVariableDataType=int8
  Header : Blocks_lib/Header  width=Portrait  addtext=''
  Selector : Selector  InputPortWidth=4  IndexOptions=Index vector (port)  Indices=[1 3]  OutputSizes=1
  Selector1 : Selector  InputPortWidth=4  IndexOptions=Index vector (port)  Indices=[1 3]  OutputSizes=1
  wires:
  N/1 -> For Iterator/1
  Vld/1 -> Selector/1
  Selector/1 -> Data Valid/Enable
  V/1 -> Selector1/1
  Selector1/1 -> Data Valid/1(V)
  For Iterator/1 -> Selector/2, Selector1/2

== system VCMGCM1962020b_v2/Fgnd/Virtual Sensors/Vehicle/Range/RangeGain/Moving Average/Subsystem ==
  In1 : Inport
  Init : Inport  Port=2
  Enable : EnablePort
  Delay : Delay  DelayLength=5  InitialConditionSource=Input port
      settings: InputPortMap=u0,p4
  Delay5 : Delay  DelayLength=10  InitialConditionSource=Input port
      settings: InputPortMap=u0,p4
  Delay6 : Delay  DelayLength=15  InitialConditionSource=Input port
      settings: InputPortMap=u0,p4
  Delay7 : Delay  DelayLength=20  InitialConditionSource=Input port
      settings: InputPortMap=u0,p4
  Out1 : Outport
  Out2 : Outport  Port=2
  Out3 : Outport  Port=3
  Out4 : Outport  Port=4
  wires:
  Delay5/1 -> Out2/1
  In1/1 -> Delay6/1, Delay7/1, Delay5/1, Delay/1
  Delay/1 -> Out1/1
  Delay7/1 -> Out4/1
  Delay6/1 -> Out3/1
  Init/1 -> Delay5/2, Delay6/2, Delay7/2, Delay/2
